simulink model "input_double"  (R2014b)
settings: Solver=ode3  SolverMode=SingleTasking  StartTime=0.0  StopTime=Tsim  FixedStep=Ts  RelTol=1e-3
InitFcn:
  | configDoubleIntegrator
values from neighbouring files (symbols this model uses):
  acc = -10    [doubleCaseTest.m]
  acc_max = 10    [doubleCaseTest.m]
  acc_min = -10    [doubleCaseTest.m]
  changeacc = -10    [doubleCaseTest.m]
  pos_init = 0    [doubleCaseTest.m]
  Ts = 0.01    [configDoubleIntegrator.m]
  vel_init = 0    [doubleCaseTest.m]
  vel_max = 100    [doubleCaseTest.m]
  vel_min = -100    [doubleCaseTest.m]
settings Model: CovMetricSettings=dwe  CovHtmlReporting=off  covSaveCumulativeToWorkspaceVar=off  CovSaveSingleToWorkspaceVar=off  CovExternalEMLEnable=on  CovSFcnEnable=on  Creator=mnade  LastModifiedBy=nina
settings DataIOCC: LimitDataPoints=off  SaveFormat=StructureWithTime
settings DebuggingCC: SolverPrmCheckMsg=none  FrameProcessingCompatibilityMsg=error  SFUnexpectedBacktrackingDiag=error  SFNoUnconditionalDefaultTransitionDiag=error
settings HardwareCC: ProdBitPerPointer=64  ProdLargestAtomicFloat=Float  ProdIntDivRoundTo=Zero  ProdEndianess=LittleEndian  ProdHWDeviceType=Specified
settings ModelReferenceCC: PropagateSignalLabelsOutOfModel=on
settings GRTTargetCC: TargetLangStandard=C99 (ISO)  GeneratePreprocessorConditionals=Use local settings

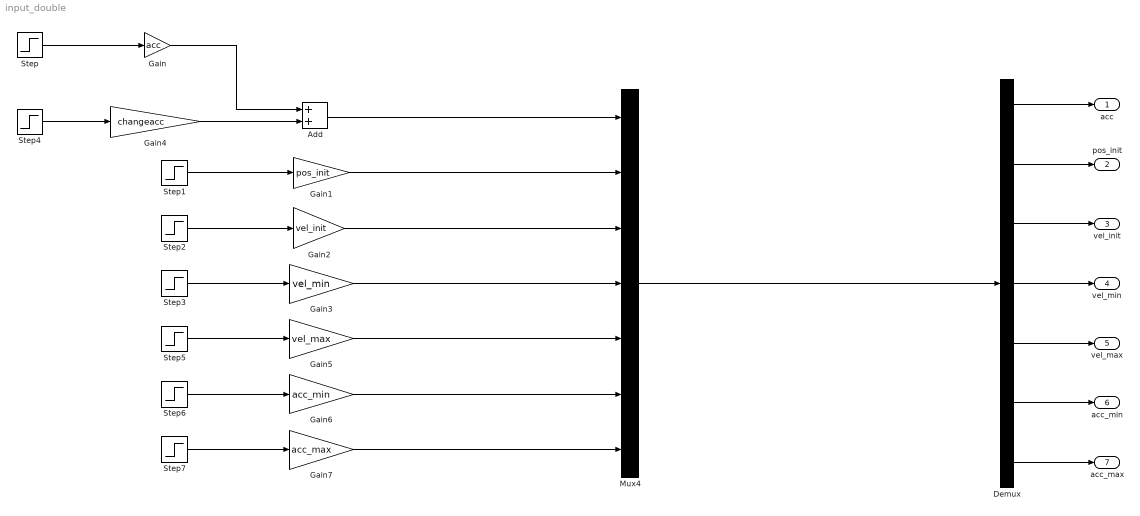
== system input_double ==
  Add : Sum
  Demux : Demux  Outputs=7
  Gain : Gain  Gain=acc
  Gain1 : Gain  Gain=pos_init
  Gain2 : Gain  Gain=vel_init
  Gain3 : Gain  Gain=vel_min
  Gain4 : Gain  Gain=changeacc
  Gain5 : Gain  Gain=vel_max
  Gain6 : Gain  Gain=acc_min
  Gain7 : Gain  Gain=acc_max
  Mux4 : Mux  Inputs=7
  Step{,1..3,5..7} (7 alike) : Step  Time=0  SampleTime=Ts
  Step4 : Step  Time=15  After=-2  SampleTime=Ts
  acc : Outport
  pos_init : Outport  Port=2
  vel_init : Outport  Port=3
  vel_min : Outport  Port=4
  vel_max : Outport  Port=5
  acc_min : Outport  Port=6
  acc_max : Outport  Port=7
  wires:
  Demux/7 -> acc_max/1
  Demux/1 -> acc/1
  Demux/2 -> pos_init/1
  Demux/3 -> vel_init/1
  Demux/4 -> vel_min/1
  Demux/5 -> vel_max/1
  Demux/6 -> acc_min/1
  Gain3/1 -> Mux4/4
  Gain2/1 -> Mux4/3
  Gain1/1 -> Mux4/2
  Step/1 -> Gain/1
  Step1/1 -> Gain1/1
  Step2/1 -> Gain2/1
  Step3/1 -> Gain3/1
  Step4/1 -> Gain4/1
  Add/1 -> Mux4/1
  Gain/1 -> Add/1
  Gain4/1 -> Add/2
  Step5/1 -> Gain5/1
  Step6/1 -> Gain6/1
  Gain6/1 -> Mux4/6
  Gain5/1 -> Mux4/5
  Step7/1 -> Gain7/1
  Gain7/1 -> Mux4/7
  Mux4/1 -> Demux/1
